simulink model "BuckConverter"  (R2023b)
settings: Solver=VariableStepAuto  StartTime=0.0  StopTime=0.01  MaxStep=1e-4  RelTol=1e-4  EnableMultiTasking=on
libraries: eeGeneralControl x4, spsCurrentMeasurementLib x2, spsSeriesRLCBranchLib x2, spsVoltageMeasurementLib x2, spsDiodeLib x1, spsMosfetLib x1, spsPWMGeneratorDCDCLib x1, simulink x1, spsVariableResistorLib x1, spsDCVoltageSourceLib x1, spspowerguiLib x1
settings Model: Creator=The MathWorks, Inc.  LastModifiedBy=prade
settings SolverCC: AlgebraicLoopSolver=TrustRegion  SolverResetMethod=Robust
settings DataIOCC: ReturnWorkspaceOutputs=off
settings OptimizationCC: EfficientFloat2IntCast=on  LifeSpan=inf
settings DebuggingCC: UnconnectedInputMsg=warning  UnconnectedOutputMsg=warning  UnconnectedLineMsg=warning  UniqueDataStoreMsg=error  StrictBusMsg=ErrorOnBusTreatedAsVector  SFUnexpectedBacktrackingDiag=warning  SFNoUnconditionalDefaultTransitionDiag=warning  SFExecutionAtInitializationDiag=none  ArithmeticOperatorsInVariantConditions=warning
settings ModelReferenceCC: EnableRefExpFcnMdlSchedulingChecks=on
settings SFSimCC: SimUseLocalCustomCode=off  CustomCodeUndefinedFunction=UseInterfaceOnly
settings RTWCC: RTWUseLocalCustomCode=off
settings CodeAppCC: StateflowObjectComments=on
settings GRTTargetCC: TargetLangStandard=C89/C90 (ANSI)
settings ConfigComp: CovMetricSettings=dw  CovSaveCumulativeToWorkspaceVar=on  CovSaveSingleToWorkspaceVar=on  CovExternalEMLEnable=off
settings SimscapeCC: SimscapeNormalizeSystem=off  SimscapeNominalValues={1, 'bar'; 1, 'cm^3/s'; 1, 'bar*kg/s'; 1, 'kJ/kg'; 1, 'kW'; }

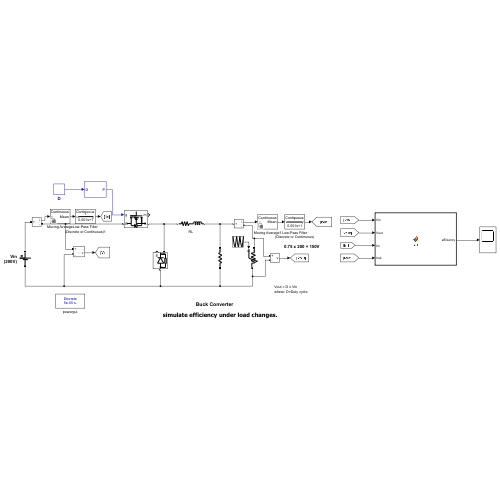
[thumbnail: Simulink's stored preview of the top-level diagram]
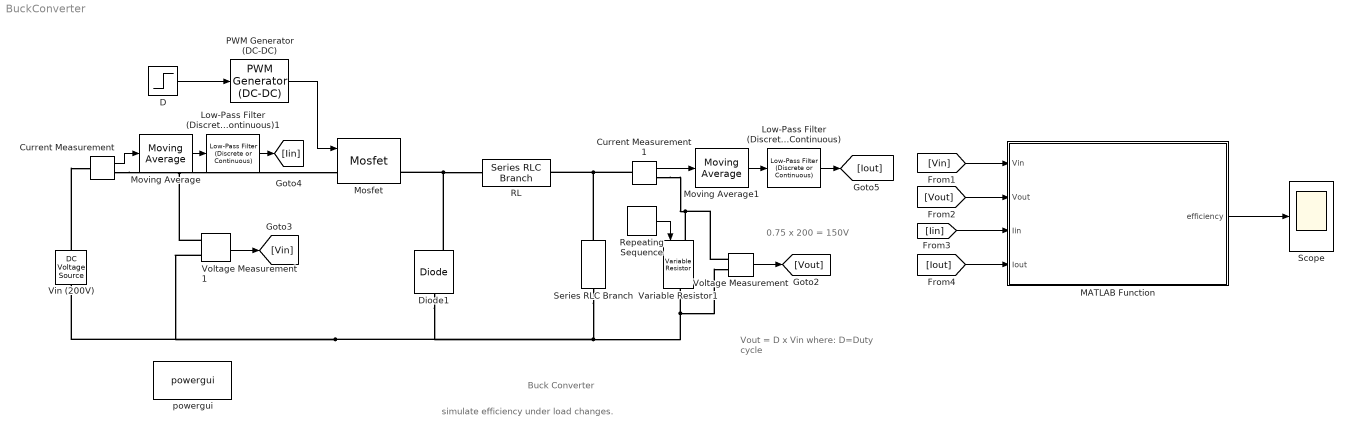
== system BuckConverter ==
  note: simulate efficiency under load changes.
  note: Vout = D x Vin
      | where: D=Duty cycle
  note: 0.75 x 200 = 150V
  note: Buck Converter
  Current Measurement : spsCurrentMeasurementLib/Current Measurement  PhasorSimulation=off  OutputType=Complex  PSBequivalent=0
  Current Measurement1 : spsCurrentMeasurementLib/Current Measurement  PhasorSimulation=off  OutputType=Complex  PSBequivalent=0
  D : Step  Time=0.0035  Before=0.5  After=0.75  SampleTime=0
  Diode1 : spsDiodeLib/Diode  Ron=0.5  Lon=0  Vf=2.5  IC=0  UseSnubber=off  Rs=1e6  Cs=1e-9  Measurements=on
  Low-Pass Filter (Discrete or Continuous) : eeGeneralControl/Low-Pass Filter (Discrete or Continuous)  K=1  T=0.001  B=inf  A=-inf  init_option=Inherited from block input  x0=0  Ts=0
  Low-Pass Filter (Discrete or Continuous)1 : eeGeneralControl/Low-Pass Filter (Discrete or Continuous)  K=1  T=0.001  B=inf  A=-inf  init_option=Inherited from block input  x0=0  Ts=0
  MATLAB Function : MATLAB Function  TreatAsAtomicUnit=on
  Mosfet : spsMosfetLib/Mosfet  Ron=1.5  Lon=0  Rd=1e-3  Vfd=4  IC=0  Rs=1e6  Cs=1e-9  Measurements=on
  Moving Average : eeGeneralControl/Moving Average  VariantControl=Variant1  LabelModeActiveChoice=Continuous  f=10e3  x0=0  BufferSize=8192  Ts=0
      settings: LibrarySourceBlock=ee_sl_lib/General Control/Moving Average
  Moving Average1 : eeGeneralControl/Moving Average  VariantControl=Variant1  LabelModeActiveChoice=Continuous  f=10e3  x0=0  BufferSize=8192  Ts=0
      settings: LibrarySourceBlock=ee_sl_lib/General Control/Moving Average
  PWM Generator (DC-DC) : spsPWMGeneratorDCDCLib/PWM Generator (DC-DC)  Fsw=10e3  Ts=0
  RL : spsSeriesRLCBranchLib/Series RLC Branch  LConnTagsString=__new0  RConnTagsString=__new0  BranchType=RL  Resistance=0.02  Inductance=3e-3  SetiL0=off  InitialCurrent=0  Capacitance=1e-6  Setx0=off  InitialVoltage=0  Measurements=None
  Repeating Sequence : simulink/Sources/Repeating Sequence  rep_seq_t=[0, 2, 4, 6, 8, 10]  rep_seq_y=[10, 5, 2, 1, 5, 10]
  Scope : Scope
  Series RLC Branch : spsSeriesRLCBranchLib/Series RLC Branch  LConnTagsString=__new0  RConnTagsString=__new0  BranchType=R  Resistance=1e8  Inductance=1e-3  SetiL0=off  InitialCurrent=0  Capacitance=1e-6  Setx0=off  InitialVoltage=0  Measurements=None
  Variable Resistor1 : spsVariableResistorLib/Variable Resistor  Rabsmin=0
      settings: LibrarySourceBlock=sps_lib/Passives/Variable Resistor
  Vin (200V) : spsDCVoltageSourceLib/DC Voltage Source  Amplitude=200  Measurements=None
  Voltage Measurement : spsVoltageMeasurementLib/Voltage Measurement  PhasorSimulation=off  OutputType=Complex  PSBequivalent=0
  Voltage Measurement1 : spsVoltageMeasurementLib/Voltage Measurement  PhasorSimulation=off  OutputType=Complex  PSBequivalent=0
  powergui : spspowerguiLib/powergui  Priority=1  SimulationMode=Discrete  SampleTime=50e-6  frequency=60  Iterations=50  frequencyindice=0  Pbase=100e6  ErrMax=1e-4  UnitsV=kV  UnitsW=MW  buscounter=0  FunctionMessages=off  echomessages=off  EnableUseOfTLC=off  CurrentSourceSwitches=off  DisableSnubberDevices=off  DisableRonSwitches=off  DisableVfSwitches=off  DisplayEquations=off  AutomaticDiscreteSolvers=off  SolverType=Tustin/Backward Euler (TBE)  Interpol=off  ExternalGateDelay=off  methode=off  Ts=100  x0status=blocks  SPID=on  SwTol=0  HookPort=off  NonlinearTolerance=1e-4  nMaxIteration=100  ContinueOnMaxIteration=off  RestoreLinks=warning  ResistiveCurrentMeasurement=off  Frange=[0:2:500]  Ylog=off  Xlog=on  ShowGrid=off  save=off  variable=ZData  structure=0  ZoomFFT=off  StartTime=0.0  cycles=1  DisplayStyle=1  fundamental=60  FreqAxis=off  MaxFrequency=1000  frequencyindicesteady=1  RmsSteady=1  display=off
  wires:
  Voltage Measurement/1 -> [Vout]
  PWM Generator (DC-DC)/1 -> Mosfet/1
  D/1 -> PWM Generator (DC-DC)/1
  Voltage Measurement1/1 -> [Vin]
  [Vin] -> MATLAB Function/1(Vin)
  [Vout] -> MATLAB Function/2(Vout)
  [Iin] -> MATLAB Function/3(Iin)
  [Iout] -> MATLAB Function/4(Iout)
  MATLAB Function/1(efficiency) -> Scope/1
  Moving Average/1 -> Low-Pass Filter (Discrete or Continuous)1/1
  Current Measurement/1 -> Moving Average/1
  Current Measurement1/1 -> Moving Average1/1
  Low-Pass Filter (Discrete or Continuous)/1 -> [Iout]
  Moving Average1/1 -> Low-Pass Filter (Discrete or Continuous)/1
  Low-Pass Filter (Discrete or Continuous)1/1 -> [Iin]
  Repeating Sequence/1 -> Variable Resistor1/1
  connections:
  Voltage Measurement1/LConn2 -- Vin (200V)/LConn1 -- Diode1/LConn1 -- Series RLC Branch/RConn1 -- Voltage Measurement/LConn2 -- Variable Resistor1/RConn1
  Current Measurement1/LConn1 -- Series RLC Branch/LConn1 -- RL/RConn1
  Voltage Measurement1/LConn1 -- Mosfet/LConn1 -- Current Measurement/RConn1
  Diode1/RConn1 -- RL/LConn1 -- Mosfet/RConn1
  Vin (200V)/RConn1 -- Current Measurement/LConn1
  Current Measurement1/RConn1 -- Variable Resistor1/LConn1 -- Voltage Measurement/LConn1

== matlab function BuckConverter/MATLAB Function ==
  data: Vin input; Vout input; Iin input; efficiency output; Iout input
function efficiency = fcn(Vin, Vout, Iin, Iout)
    Pin = Vin * Iin;
    Pout = Vout * Iout;
    if Pin > 0
        efficiency = (Pout / Pin) * 100;
    else
        efficiency = 0;
    end
    % Limit to realistic range
    efficiency = max(0, min(100, efficiency));
end
